simulink model "Cascaded_H_Bridge_Multilevel_Inverter"  (R2024a)
settings: Solver=FixedStepAuto  StartTime=0.0  StopTime=200/fe  FixedStep=1/(100*fsw)  RelTol=1e-3
values from neighbouring files (symbols this model uses):
  B = 0*0.0025    (= 0)    [ECE_598_script_file.m]
  fe = 100    [ECE_598_script_file.m]
  fsw = 1000    [ECE_598_script_file.m]
  J = 0.01    [ECE_598_script_file.m]
  Lrl_dash = 9.6e-3    (= 0.0096)    [ECE_598_script_file.m]
  Lsl = 9.6e-3    (= 0.0096)    [ECE_598_script_file.m]
  M = 165e-3    (= 0.165)    [ECE_598_script_file.m]
  Rr = 4.23    [ECE_598_script_file.m]
  Rs = 3.57    [ECE_598_script_file.m]
  tau_L = 2    [ECE_598_script_file.m]
  turns_ratio = 0.682    [ECE_598_script_file.m]
  Vdc = 400    [ECE_598_script_file.m]
  Vm = 200    [ECE_598_script_file.m]
undefined symbols (not defined in the file or in its folder): j, jsin
libraries: nesl_utility x22, ee_lib x15, fl_lib x11
(part 2 of 2)

== matlab function Cascaded_H_Bridge_Multilevel_Inverter/Switching Signal Generator/MATLAB Function ==
  data: Vref input; q11 output; time input; fsw input; sorted_switching_seq input; sorted_time_switching_seq input; q12 output; q13 output; q14 output; q21 output; q22 output; q23 output; q24 output; q31 output; q32 output; q33 output; q34 output; sorted_switching_seq output; sorted_time_switching_seq output
function [q11, q12, q13, q14, q21, q22, q23, q24, q31, q32, q33, q34, sorted_switching_seq, sorted_time_switching_seq] = fcn(Vref, time, fsw, sorted_switching_seq, sorted_time_switching_seq)

% fprintf('actual cycle = %.2f / fsw \n',time*fsw);
% fprintf('mod value at time = %.5f sec (time, 1/fsw) = %.20f compare between %.20f and %.20f \n', time, mod(time*fsw,1), 1e-10, 1-1e-10);
% fprintf(' boolean value = %d \n',int32((mod(time*fsw,1) < 1e-10 && mod(time*fsw,1) > 0) || (mod(time*fsw,1) > 1-1e-10 && mod(time*fsw,1) < 1)));


% fe = 10;

% disp(mod(time, 1/(10*fe)))

% if (mod(time*fe*10, 1) < 1e-7)
%     Vref_angle = angle(Vref)*180/pi;
% 
%     fprintf('time = %.5f us',time)
%     fprintf('cycle period = %.2f / fe',mod(time,1/fe))
%     fprintf('angle = %.2f degree',Vref_angle)
%     disp('sorted switching seq :')
%     disp(sorted_switching_seq)
%     disp('In here !!!!!!!!!!!!!!!!!!!!!!!!!!!')
% 
% end

% if (time > 0.24)
%     fprintf('time = %.5f / fsw \n',time*fsw);
%     fprintf('value of mod(time*fsw,1) = %.20f \n',mod(time*fsw,1));
% end


if (time == 0)
    sorted_switching_seq = zeros(6,3);
    sorted_time_switching_seq = zeros(6,1);

    q11 = -100;
    q12 = 100;
    q13 = -100;
    q14 = 100;

    q21 = -100;
    q22 = 100;
    q23 = -100;
    q24 = 100;

    q31 = -100;
    q32 = 100;
    q33 = -100;
    q34 = 100;





elseif((mod(time*fsw,1) < 10e-5 && mod(time*fsw,1) > 0) || (mod(time*fsw,1) > 1-10e-5 && mod(time*fsw,1) < 1))
    
    % disp('sorted switching seq before start of loop = ')
    % disp(sorted_switching_seq)
    % fprintf('In here at time = %.5f \n',time);
    % fprintf('Value of mod = %.20f \n',mod(time*fsw,1));
    %%  Inputs for 3-level inverter (all types)
    
    % fsw = 200; %1e3;                                                               % Switching frequency (Hz)
    fe = 10; %100;                                                                   % sine frequency (Hz)
    % Vm = 400;                                                                  % input voltage peak (V)
    Vdc = 400/2;                                                                 % Input DC voltage (V)

    %% Defining ref vector values

    ref_vec_vals = zeros(19, 3, 3);
    
    % Zero vectors
    % ref_vec_vals(1, :, :) = reshape(transpose([0,0,0 ; -1, -1, -1 ; 1, 1, 1]), 1, 3, []);
    ref_vec_vals(1, :, 1:2) = reshape(transpose([-1, -1, -1 ; 1, 1, 1]), 1, 3, []);
    
    %  Outer sector vectors / medium and large vectors
    ref_vec_vals(2, :, 1) = reshape(transpose([1, -1, -1]),1,3,[]);
    ref_vec_vals(3, :, 1) = reshape(transpose([1, 0, -1]), 1, 3, []);
    ref_vec_vals(4, :, 1) = reshape(transpose([1, 1, -1]),1,3,[]);
    ref_vec_vals(5, :, 1) = reshape(transpose([0, 1, -1]),1,3,[]);
    ref_vec_vals(6, :, 1) = reshape(transpose([-1, 1, -1]),1,3,[]);
    ref_vec_vals(7, :, 1) = reshape(transpose([-1, 1, 0]),1,3,[]);
    ref_vec_vals(8, :, 1) = reshape(transpose([-1, 1, 1]),1,3,[]);
    ref_vec_vals(9, :, 1) = reshape(transpose([-1, 0, 1]),1,3,[]);
    ref_vec_vals(10, :, 1) = reshape(transpose([-1, -1, 1]),1,3,[]);
    ref_vec_vals(11, :, 1) = reshape(transpose([0, -1, 1]),1,3,[]);
    ref_vec_vals(12, :, 1) = reshape(transpose([1, -1, 1]),1,3,[]);
    % ref_vec_vals(13, :, 1) = reshape(transpose([1, -1, 1]),1,3,[]);
    ref_vec_vals(13, :, 1) = reshape(transpose([1, -1, 0]),1,3,[]);
    
    % Inner circle vectors / small vectors
    ref_vec_vals(14, :, 1:2) = reshape(transpose([1, 0, 0 ; 0, -1, -1]),1,3,[]);
    ref_vec_vals(15, :, 1:2) = reshape(transpose([1, 1, 0 ; 0, 0, -1]),1,3,[]);
    ref_vec_vals(16, :, 1:2) = reshape(transpose([0, 1, 0 ; -1, 0, -1]),1,3,[]);
    ref_vec_vals(17, :, 1:2) = reshape(transpose([0, 1, 1 ; -1, 0, 0]),1,3,[]);
    ref_vec_vals(18, :, 1:2) = reshape(transpose([0, 0, 1 ; -1, -1, 0]),1,3,[]);
    ref_vec_vals(19, :, 1:2) = reshape(transpose([1, 0, 1 ; 0, -1, 0]),1,3,[]);

    ref_vec_vals(14, :, 1:2) = reshape(transpose([1, 0, 0 ; 0, -1, -1]),1,3,[]);
    ref_vec_vals(15, :, 1:2) = reshape(transpose([0, 0, -1 ; 1, 1, 0 ]),1,3,[]);
    ref_vec_vals(16, :, 1:2) = reshape(transpose([0, 1, 0 ; -1, 0, -1]),1,3,[]);
    ref_vec_vals(17, :, 1:2) = reshape(transpose([-1, 0, 0 ; 0, 1, 1 ]),1,3,[]);
    ref_vec_vals(18, :, 1:2) = reshape(transpose([0, 0, 1 ; -1, -1, 0]),1,3,[]);
    ref_vec_vals(19, :, 1:2) = reshape(transpose([0, -1, 0 ; 1, 0, 1 ]),1,3,[]);
    
    %% Defing ref vectors
    
    ref_vecs = complex(zeros(19, 1));
    
    % Zero vector 
    ref_vecs(1) = 0 + 0j;
    
    % Outer sector vectors / medium and large vectors
    for i = 1:12
        if mod(i,2) == 0
            x = i/2;
            ang = 30 + 60*(x-1);
            ref_vecs(i+1) = sqrt(3)*Vdc*exp(1j*ang*pi/180);
        else 
            x = (i+1)/2;
            ang = 60*(x-1);
            ref_vecs(i+1) = 2*Vdc*exp(1j*ang*pi/180);
        end
    end
    
    
    % Inner sector vectors / small vectors
    for i = 1:6
        ang = 60*(i-1);
        ref_vecs(i+13) = Vdc*exp(1j*ang*pi/180);
    end
    
    
    %% Defining Main Sector vectors
    
    sector_vecs = zeros(6, 7);
    
    sector_vecs(1,:) = [14, 1, 2, 15, 0, 19, 12];
    sector_vecs(2,:) = [15, 2, 3, 4, 16, 0, 14];
    sector_vecs(3,:) = [16, 15, 4, 5, 6, 17, 0];
    sector_vecs(4,:) = [17, 0, 16, 6, 7, 8, 18];
    sector_vecs(5,:) = [18, 19, 0, 17, 8, 9, 10];
    sector_vecs(6,:) = [19, 13, 14, 0, 18, 10, 11];
    
    
    
    sector_vecs(1,:) = [14, 2, 3, 15, 1, 19, 13];
    sector_vecs(2,:) = [15, 3, 4, 5, 16, 1, 14];
    sector_vecs(3,:) = [16, 15, 5, 6, 7, 17, 1];
    sector_vecs(4,:) = [17, 1, 16, 7, 8, 9, 18];
    sector_vecs(5,:) = [18, 19, 1, 17, 9, 10, 11];
    sector_vecs(6,:) = [19, 13, 14, 1, 18, 11, 12];


    %% defining variables

    index_final_vecs = zeros(3);
    final_vecs = zeros(3);
    final_vecs_phase = zeros(3);
    final_vecs_mag = zeros(3);


    angle_vec = angle(Vref); 
    phase = mod(angle_vec, 2*pi).*(180/pi);
    
    
    main_sec_index = -1;
    
    if (phase >= 0 && phase < 30) || (phase >= 330 && phase <= 360)
        main_sec_index = 1;
    
    elseif phase >= 30 && phase < 90
        main_sec_index = 2;
    
    elseif phase >= 90 && phase < 150
        main_sec_index = 3;
    
    elseif phase >= 150 && phase < 210
        main_sec_index = 4;
    
    elseif phase >= 210 && phase < 270
        main_sec_index = 5;
    
    elseif phase >= 270 && phase < 330
        main_sec_index = 6;
    
    else 
        error('vec does not lie within 0 to 360 degree');
    end
    
    %% Working inside the main sector
    
    vec_ref_to_sec = Vref - ref_vecs(sector_vecs(main_sec_index,1));
    
    vec_1 = ref_vecs(sector_vecs(main_sec_index,2)) - ref_vecs(sector_vecs(main_sec_index,1));
    vec_2 = ref_vecs(sector_vecs(main_sec_index,3)) - ref_vecs(sector_vecs(main_sec_index,1));
    vec_3 = ref_vecs(sector_vecs(main_sec_index,4)) - ref_vecs(sector_vecs(main_sec_index,1));
    vec_4 = ref_vecs(sector_vecs(main_sec_index,5)) - ref_vecs(sector_vecs(main_sec_index,1));
    vec_5 = ref_vecs(sector_vecs(main_sec_index,6)) - ref_vecs(sector_vecs(main_sec_index,1));
    vec_6 = ref_vecs(sector_vecs(main_sec_index,7)) - ref_vecs(sector_vecs(main_sec_index,1));
    
    
    angle_dash = angle(vec_ref_to_sec); 
    
    phase_dash = mod(angle_dash, 2*pi).*(180/pi);
    
    
    final_vec_index = zeros(2);
    
    sub_sec_index = -1;
    
    if (phase_dash >= 0 && phase_dash < 60) 
        sub_sec_index = 1;
        final_vec_index(1) = sector_vecs(main_sec_index,2);
        final_vec_index(2) = sector_vecs(main_sec_index,3);
    
    elseif phase_dash >= 60 && phase_dash < 120
        sub_sec_index = 2;
        final_vec_index(1) = sector_vecs(main_sec_index,3);
        final_vec_index(2) = sector_vecs(main_sec_index,4);
    
    elseif phase_dash >= 120 && phase_dash < 180
        sub_sec_index = 3;
        final_vec_index(1) = sector_vecs(main_sec_index,4);
        final_vec_index(2) = sector_vecs(main_sec_index,5);
    
    elseif phase_dash >= 180 && phase_dash < 240
        sub_sec_index = 4;
        final_vec_index(1) = sector_vecs(main_sec_index,5);
        final_vec_index(2) = sector_vecs(main_sec_index,6);
    
    elseif phase_dash >= 240 && phase_dash < 300
        sub_sec_index = 5;
        final_vec_index(1) = sector_vecs(main_sec_index,6);
        final_vec_index(2) = sector_vecs(main_sec_index,7);
    
    elseif phase_dash >= 300 && phase_dash <= 360
        sub_sec_index = 6;
        final_vec_index(1) = sector_vecs(main_sec_index,7);
        final_vec_index(2) = sector_vecs(main_sec_index,2);
    
    else 
        error('vec does not lie within 0 to 360 degree');
    end
    
    final_vec_index(3) = sector_vecs(main_sec_index,1);
    
    index_final_vecs = [final_vec_index(1), final_vec_index(2), final_vec_index(3)];

    num_of_small_vecs = 0;
    for iter = 1:3
        if (index_final_vecs(iter) >= 14 && index_final_vecs(iter) <= 19)
            num_of_small_vecs = num_of_small_vecs + 1;
        end
    end

    vec1 = ref_vecs(final_vec_index(1));
    vec2 = ref_vecs(final_vec_index(2));
    vec3 = ref_vecs(final_vec_index(3));
    
    final_vecs = [vec1, vec2, vec3];
    final_vecs_phase = angle(final_vecs(:));
    final_vecs_mag = abs(final_vecs(:));

    
    %% Finding time durations
    phase = angle(Vref);
    magnitude = abs(Vref);
    
    A_matrix = [final_vecs_mag(1)*cos(final_vecs_phase(1)), final_vecs_mag(2)*cos(final_vecs_phase(2)), final_vecs_mag(3)*cos(final_vecs_phase(3));
                    final_vecs_mag(1)*sin(final_vecs_phase(1)), final_vecs_mag(2)*sin(final_vecs_phase(2)), final_vecs_mag(3)*sin(final_vecs_phase(3));
                    1,                          1,                          1];
        
    
    B_matrix = [(magnitude*cos(phase))*(1/fsw); magnitude*sin(phase)*(1/fsw); (1/fsw)];
    
    T_values = inv(A_matrix)*B_matrix;
    
    % final_T_vals(i,1) = T_values(1);
    % final_T_vals(i,2) = T_values(2);
    % final_T_vals(i,3) = T_values(3);

    T1 = T_values(1);
    T2 = T_values(2);
    T3 = T_values(3);
    
    
    %% Defining the switching states of 
    
    % 1) q11, q12, q13, q14
    % 2) q21, q22, q23, q24
    % 3) q31, q32, q33, q34
    
    % stored_values = zeros(6,3);

    % switching_seq = zeros(2*num_of_small_vecs + (3-num_of_small_vecs), 3);
    % time_switching_seq = zeros(2*num_of_small_vecs + (3-num_of_small_vecs), 1);


    % Finding out the number of small vectors

    % count_small_vectors = 0;
    % small_vec_index = zeros(3,1);
    % small_vec_index_time = zeros(3,1);
    T_value_last = 0;
    index_last = 100;

    permission_for_split = ones(3,1);

    for iter_small=1:length(index_final_vecs)
        if (index_final_vecs(iter_small) > 13)
            % count_small_vectors = count_small_vectors + 1;
            % small_vec_index(iter_count_small_vecs) = index_final_vecs(iter_count_small_vecs);
            % small_vec_index_time(iter_count_small_vecs) = T_values(iter_count_small_vecs);
            if (T_value_last == 0)
                T_value_last = T_values(iter_small);
                index_last = iter_small;
                permission_for_split(iter_small) = 1;
            else
                if (T_values(iter_small) > T_value_last)
                    permission_for_split(iter_small) = 1;
                    permission_for_split(index_last) = 0;

                    T_value_last = T_values(iter_small);
                    index_last = iter_small;
                else
                    permission_for_split(iter_small) = 0;
                end
            end
        end
    end
    
    % fprintf('time = %.5f \n',time);
    % disp('Vec indices = ');
    % disp(index_final_vecs);
    % disp('associated times = ');
    % disp(T_values);
    % disp('permission to split = ');
    % disp(permission_for_split);
    % disp(' ')

    switching_seq = 100*ones(6,3);
    time_switching_seq = (1/fsw)*ones(6,1);
    
    count = 0;
    for iter = 1:length(index_final_vecs)
        index = index_final_vecs(iter);

        % if (index < 14)
        %     permission_for_split(iter) = 0;                                 % if not small vector, make this variable temporarily vanish in the if statements
        % end

        count = count + 1;
        switching_seq(count, :) = ref_vec_vals(index,:,1);
    
        if (ref_vec_vals(index,1,2) == 0 && ref_vec_vals(index,2,2) == 0 && ref_vec_vals(index,3,2) == 0 || permission_for_split(iter) == 0)
            time_switching_seq(count) = T_values(iter);
            continue
        end
    
        count = count + 1;
        
        % disp('vec values : ');
        % disp(ref_vec_vals(index,:,2));
        % fprintf('\n permission to plit = %.1f \n',permission_for_split(iter));
        % fprintf('iter = %.1f \n',iter);
        % fprintf('count = %.1f \n',count);

        switching_seq(count, :) = ref_vec_vals(index,:,2);
    
        if (ref_vec_vals(index,1,3) == 0 && ref_vec_vals(index,2,3) == 0 && ref_vec_vals(index,3,3) == 0 || permission_for_split(iter) == 0)
            time_switching_seq(count-1) = T_values(iter)/2;
            time_switching_seq(count) = T_values(iter)/2;
            continue
        end
    
        count = count + 1;
        switching_seq(count, :) = ref_vec_vals(index,:,3);

        time_switching_seq(count-2) = T_values(iter)/3;
        time_switching_seq(count-1) = T_values(iter)/3;
        time_switching_seq(count) = T_values(iter)/3;
        
    end

    % Step 1: Compute row sums
    row_sums = sum(switching_seq, 2);  % This is a 6x1 column vector
    
    % Step 2: Get sorting index based on row sums
    [~, sort_idx] = sort(row_sums, 'ascend');
    
    % disp('unsorted switching seq end of loop :')
    % disp(switching_seq)

    % Step 3: Reorder the rows using the index
    sorted_switching_seq = switching_seq(sort_idx, :);
    sorted_time_switching_seq = time_switching_seq(sort_idx);
    

    if (time > 0)
        angle_Vref = angle(Vref)*180/pi;
        % fprintf('cycle = %.3f / fsw \n',time*fsw);
        % fprintf('time = %.5f \n',time);
        % fprintf('cycle = %.3f / fe = \n',time*fe);
        % fprintf('angle = %.3f \n',angle_Vref);
        % fprintf('main sec = %.1f and sub_sec index = %.1f \n',main_sec_index,sub_sec_index);
        % disp('sorted switching seq : ');
        % disp(sorted_switching_seq);
        % disp(' ');
        % disp('sorted time seq : ');
        % disp(sorted_time_switching_seq);
        % disp(' ')
    end
    
    % disp('sorted switching seq end of loop :');
    % disp(sorted_switching_seq);
    % disp('sorted time switching seq :');
    % disp(time_switching_seq.*1e6);
    
    % disp('sorted switching seq :')
    % disp(sorted_switching_seq);
    % disp('sorted time switching seq :')
    % disp(sorted_time_switching_seq.*1e6)
    % disp([sprintf('T1 = %.2f us', T1*1e6)])
    % disp([sprintf('T2 = %.2f us', T2*1e6)])
    % disp([sprintf('T3 = %.2f us', T3*1e6)])


    switch_seq = sorted_switching_seq(1,:);

    % disp('switch_seq = ')
    % disp(switch_seq)


    if (switch_seq(1) == 1)
        q11 = 100;
        q12 = 100;
        q13 = -100;
        q14 = -100;

    elseif (switch_seq(1) == -1)

        q11 = -100;
        q12 = -100;
        q13 = 100;
        q14 = 100;

    else
        q11 = -100;
        q12 = 100;
        q13 = -100;
        q14 = 100;
    end


    if (switch_seq(2) == 1)
        q21 = 100;
        q22 = 100;
        q23 = -100;
        q24 = -100;

    elseif (switch_seq(2) == -1)

        q21 = -100;
        q22 = -100;
        q23 = 100;
        q24 = 100;

    else
        q21 = -100;
        q22 = 100;
        q23 = -100;
        q24 = 100;
    end


    if (switch_seq(3) == 1)
        q31 = 100;
        q32 = 100;
        q33 = -100;
        q34 = -100;

    elseif (switch_seq(3) == -1)

        q31 = -100;
        q32 = -100;
        q33 = 100;
        q34 = 100;

    else
        q31 = -100;
        q32 = 100;
        q33 = -100;
        q34 = 100;
    end

else
    sub_time = mod(time,(1/fsw));
    
    % disp([sprintf('time = %.2f us', time*1e6)])
    % disp([sprintf('sub_time = %.2f us', sub_time*1e6)])
    % 
    % for i = 1:length(sorted_time_switching_seq)
    %     fprintf('T_%d = %.2f\n', int32(i), sorted_time_switching_seq(i)*1e6);
    % end
    dummy_var = 0;
    for iter = 1:6
        if (sorted_time_switching_seq(iter) ~= 1/fsw)
            dummy_var = dummy_var + sorted_time_switching_seq(iter)/2;
        end
    end
  

    if (0 <= sub_time && sub_time <= sorted_time_switching_seq(1)/2 && sorted_time_switching_seq(1) ~= 1/fsw)
        switch_seq = sorted_switching_seq(1,:);
    
    elseif (sorted_time_switching_seq(1)/2 <= sub_time && sub_time <= sorted_time_switching_seq(1)/2 + sorted_time_switching_seq(2)/2 && sorted_time_switching_seq(2) ~= 1/fsw)
        switch_seq = sorted_switching_seq(2,:);

    elseif ((sorted_time_switching_seq(1)/2 + sorted_time_switching_seq(2)/2) <= sub_time && sub_time <= (sorted_time_switching_seq(1)/2 + sorted_time_switching_seq(2)/2 + sorted_time_switching_seq(3)/2) && sorted_time_switching_seq(3) ~= 1/fsw)
        switch_seq = sorted_switching_seq(3,:);
    
    elseif ((sorted_time_switching_seq(1)/2 + sorted_time_switching_seq(2)/2 + sorted_time_switching_seq(3)/2) <= sub_time && sub_time <= (sorted_time_switching_seq(1)/2 + sorted_time_switching_seq(2)/2 + sorted_time_switching_seq(3)/2 + sorted_time_switching_seq(4)/2) && sorted_time_switching_seq(4) ~= 1/fsw)
        switch_seq = sorted_switching_seq(4,:);

    elseif ((sorted_time_switching_seq(1)/2 + sorted_time_switching_seq(2)/2 + sorted_time_switching_seq(3)/2 + sorted_time_switching_seq(4)/2) <= sub_time && sub_time <= (sorted_time_switching_seq(1)/2 + sorted_time_switching_seq(2)/2 + sorted_time_switching_seq(3)/2 + sorted_time_switching_seq(4)/2 + sorted_time_switching_seq(5)/2) && sorted_time_switching_seq(5) ~= 1/fsw)
        switch_seq = sorted_switching_seq(5,:);

    elseif ((sorted_time_switching_seq(1)/2 + sorted_time_switching_seq(2)/2 + sorted_time_switching_seq(3)/2 + sorted_time_switching_seq(4)/2 + sorted_time_switching_seq(5)/2) <= sub_time && sub_time <= (sorted_time_switching_seq(1)/2 + sorted_time_switching_seq(2)/2 + sorted_time_switching_seq(3)/2 + sorted_time_switching_seq(4)/2 + sorted_time_switching_seq(5)/2 + sorted_time_switching_seq(6)/2) && sorted_time_switching_seq(6) ~= 1/fsw)
        switch_seq = sorted_switching_seq(6,:);
    


    % 
    % disp('Value 1 = ')
    % disp((2*dummy_var - (sorted_time_switching_seq(1)/2 + sorted_time_switching_seq(2)/2 + sorted_time_switching_seq(3)/2 + sorted_time_switching_seq(4)/2 + sorted_time_switching_seq(5)/2)) <= sub_time)
    % disp('Value 2 = ')
    % disp(sub_time <= (2*dummy_var - (sorted_time_switching_seq(1)/2 + sorted_time_switching_seq(2)/2 + sorted_time_switching_seq(3)/2 + sorted_time_switching_seq(4)/2)))
    % disp('Value 3 = ')
    % disp(sorted_time_switching_seq(6) ~= 1/fsw)




    % corrected reverse
    elseif (2*dummy_var - (sorted_time_switching_seq(1)/2 + sorted_time_switching_seq(2)/2 + sorted_time_switching_seq(3)/2 + sorted_time_switching_seq(4)/2 + sorted_time_switching_seq(5)/2 + sorted_time_switching_seq(6)/2)) <= sub_time && sub_time <= (2*dummy_var - (sorted_time_switching_seq(1)/2 + sorted_time_switching_seq(2)/2 + sorted_time_switching_seq(3)/2 + sorted_time_switching_seq(4)/2 + sorted_time_switching_seq(5)/2)) && sorted_time_switching_seq(6) ~= 1/fsw
        switch_seq = sorted_switching_seq(6,:);

    elseif (2*dummy_var - (sorted_time_switching_seq(1)/2 + sorted_time_switching_seq(2)/2 + sorted_time_switching_seq(3)/2 + sorted_time_switching_seq(4)/2 + sorted_time_switching_seq(5)/2)) <= sub_time && sub_time <= (2*dummy_var - (sorted_time_switching_seq(1)/2 + sorted_time_switching_seq(2)/2 + sorted_time_switching_seq(3)/2 + sorted_time_switching_seq(4)/2)) && sorted_time_switching_seq(5) ~= 1/fsw
        switch_seq = sorted_switching_seq(5,:);

    elseif (2*dummy_var - (sorted_time_switching_seq(1)/2 + sorted_time_switching_seq(2)/2 + sorted_time_switching_seq(3)/2 + sorted_time_switching_seq(4)/2)) <= sub_time && sub_time <= (2*dummy_var - (sorted_time_switching_seq(1)/2 + sorted_time_switching_seq(2)/2 + sorted_time_switching_seq(3)/2)) && sorted_time_switching_seq(4) ~= 1/fsw
        switch_seq = sorted_switching_seq(4,:);

    elseif (2*dummy_var - (sorted_time_switching_seq(1)/2 + sorted_time_switching_seq(2)/2 + sorted_time_switching_seq(3)/2)) <= sub_time && sub_time <= (2*dummy_var - (sorted_time_switching_seq(1)/2 + sorted_time_switching_seq(2)/2)) && sorted_time_switching_seq(3) ~= 1/fsw
        switch_seq = sorted_switching_seq(3,:);

    elseif (2*dummy_var - (sorted_time_switching_seq(1)/2 + sorted_time_switching_seq(2)/2)) <= sub_time && sub_time <= (2*dummy_var - (sorted_time_switching_seq(1)/2)) && sorted_time_switching_seq(2) ~= 1/fsw
        switch_seq = sorted_switching_seq(2,:);

    elseif (2*dummy_var - (sorted_time_switching_seq(1)/2)) <= sub_time && sub_time <= (2*dummy_var - 0) && sorted_time_switching_seq(1) ~= 1/fsw
        switch_seq = sorted_switching_seq(1,:);

    else 
        switch_seq = [0, 0, 0];
        % error('sub_time goin above limit !')
    end
    
    % fprintf('sub_time = %.2f us\n',sub_time*1e6);
    % disp('switch seq : ')
    % disp(switch_seq)

        
    if (switch_seq(1) == 1)
        q11 = 100;
        q12 = 100;
        q13 = -100;
        q14 = -100;

    elseif (switch_seq(1) == -1)

        q11 = -100;
        q12 = -100;
        q13 = 100;
        q14 = 100;

    else
        q11 = -100;
        q12 = 100;
        q13 = -100;
        q14 = 100;
    end


    if (switch_seq(2) == 1)
        q21 = 100;
        q22 = 100;
        q23 = -100;
        q24 = -100;

    elseif (switch_seq(2) == -1)

        q21 = -100;
        q22 = -100;
        q23 = 100;
        q24 = 100;

    else
        q21 = -100;
        q22 = 100;
        q23 = -100;
        q24 = 100;
    end


    if (switch_seq(3) == 1)
        q31 = 100;
        q32 = 100;
        q33 = -100;
        q34 = -100;

    elseif (switch_seq(3) == -1)

        q31 = -100;
        q32 = -100;
        q33 = 100;
        q34 = 100;

    else
        q31 = -100;
        q32 = 100;
        q33 = -100;
        q34 = 100;
    end

    
end
